simulink model "torqueControlBalancing"  (Simulink 9.1)
settings: Solver=FixedStepDiscrete  StartTime=0.0  StopTime="Config.SIMULATION_TIME "  FixedStep=Config.tStep  RelTol=1e-3  EnableMultiTasking=on
PostLoadFcn:
  | %% Try to open the static GUI and try to adjust it
  | try
  | 
  |     staticGUI = simulinkStaticGUI;
  | 
  | end
InitFcn:
  | %% initialize the simulation
  | cd(fileparts(which(bdroot)));
  | initTorqueControlBalancing;
  | 
  | %% Try to edit the GUI (the user may have already closed it)
  | try
  | 
  |     %% Update Start Button
  |     set(sl_synch_handles.startButton,'Backgroundcolor',[0.0,1.0,0.0]);
  |     set(sl_synch_handles.startButton,'Enable','on');
  | 
  | end
StartFcn:
  | %% Try to edit the GUI (the user may have already closed it)
  | try
  | 
  |     %% Update Start Button
  |     set(sl_synch_handles.startButton,'Backgroundcolor',[0.8,0.8,0.8]);
  |     set(sl_synch_handles.startButton,'Enable','off');
  | 
  |     %% Update Compile Button
  |     set(sl_synch_handles.compileButton,'Backgroundcolor',[0.8,0.8,0.8]);
  |     set(sl_synch_handles.compileButton,'Enable','off');
  | 
  |     %% Update Exit Button
  |     set(sl_synch_handles.exitButton,'Backgroundcolor',[0.8,0.8,0.8]);
  |     set(sl_synch_handles.exitButton,'Enable','off');
  | 
  | end
StopFcn:
  | %% stop the simulation
  | cd(fileparts(which(bdroot)));
  | stopTorqueControlBalancing;
  | 
  | %% Try to edit the GUI (the user may have already closed it)
  | try
  | 
  |     %% Update Compile Button
  |     set(sl_synch_handles.compileButton,'Backgroundcolor',[1.0,0.6,0.0]);
  |     set(sl_synch_handles.compileButton,'Enable','on');
  | 
  |     %% Update Exit Button
  |     set(sl_synch_handles.exitButton,'Backgroundcolor',[0.0,1.0,1.0]);
  |     set(sl_synch_handles.exitButton,'Enable','on');
  | 
  | end
undefined symbols (not defined in the file or in its folder): bVectorConstraints, Config, ConstraintsMatrix, Gain, Reg, ROBOT_DOF, Sat, StateMachine
libraries: WBToolboxLibrary x77
(part 1 of 2)
CloseFcn:
  | %% Try to close the GUI (the user might have already closed it)
  | try
  | 
  |     close(simulinkStaticGUI)
  | 
  | end
settings Model: SuppressorTable=22 serialization::archive 11 0 6 0 0 0 0 0  Creator=daniele  LastModifiedBy=lrapetti
settings DataIOCC: LimitDataPoints=on
settings OptimizationCC: ExpressionDepthLimit=2147483647
settings DebuggingCC: SolverPrmCheckMsg=warning  FcnCallInpInsideContextMsg=warning  AllowSymbolicDim=off  StateNameClashWarn=warning
settings SFSimCC: SimParseCustomCode=off
settings RTWCC: GenCodeOnly=on  TargetLang=C++
settings GRTTargetCC: TargetLangStandard=C++03 (ISO)  GeneratePreprocessorConditionals=Disable all  CombineOutputUpdateFcns=on  MatFileLogging=off  MultiInstanceERTCode=on  CodeInterfacePackaging=C++ class  SupportNonFinite=off  GRTInterface=off
settings CPPComponent: GenerateDestructor=on  GenerateExternalIOAccessMethods=None  ParameterMemberVisibility=private  InternalMemberVisibility=private  GenerateParameterAccessMethods=None  GenerateInternalMemberAccessMethods=None  UseOperatorNewForModelRefRegistration=off

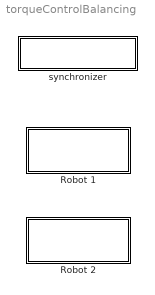
== system torqueControlBalancing ==
  Robot 1 : Subsystem
  Robot 2 : Subsystem
  synchronizer : Subsystem
      mask Display: disp('SYNCHRONIZER')

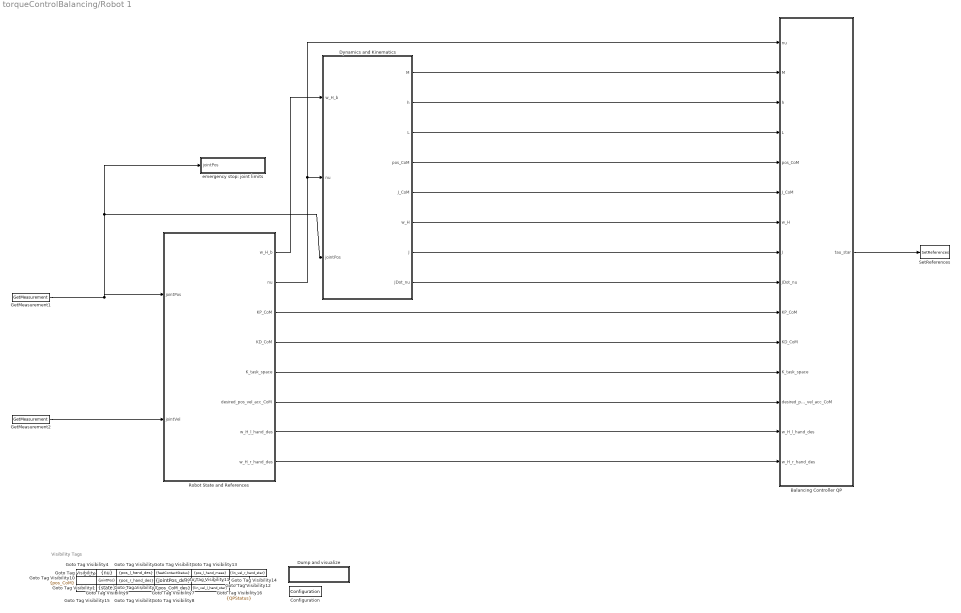
== system torqueControlBalancing/Robot 1 ==
  note: Visibility Tags
  Balancing Controller QP : Subsystem
  Configuration : WBToolboxLibrary/Utilities/Configuration  ConfigSource=Workspace  ConfigObject='WBTConfigRobot_1'
      settings: SourceProductName=WholeBodyToolbox
  Dump and visualize : Subsystem
      mask Display: disp('VISUALIZER')
  Dynamics and Kinematics : Subsystem
  GetMeasurement1 : WBToolboxLibrary/States/GetMeasurement  measuredType=Joints Position
      settings: SourceProductName=WholeBodyToolbox
  GetMeasurement2 : WBToolboxLibrary/States/GetMeasurement  measuredType=Joints Velocity
      settings: SourceProductName=WholeBodyToolbox
  Goto Tag Visibility : GotoTagVisibility  GotoTag=nu
  Goto Tag Visibility1 : GotoTagVisibility  GotoTag=state
  Goto Tag Visibility10 : GotoTagVisibility  GotoTag=pos_CoM
  Goto Tag Visibility11 : GotoTagVisibility  GotoTag=lin_vel_l_hand_star
  Goto Tag Visibility12 : GotoTagVisibility  GotoTag=lin_vel_r_hand_star
  Goto Tag Visibility13 : GotoTagVisibility  GotoTag=pos_l_hand_meas
  Goto Tag Visibility14 : GotoTagVisibility  GotoTag=pos_r_hand_meas
  Goto Tag Visibility15 : GotoTagVisibility  GotoTag=tau_star
  Goto Tag Visibility16 : GotoTagVisibility  GotoTag=QPStatus
  Goto Tag Visibility2 : GotoTagVisibility  GotoTag=pos_l_hand_des
  Goto Tag Visibility3 : GotoTagVisibility  GotoTag=pos_r_hand_des
  Goto Tag Visibility4 : GotoTagVisibility  GotoTag=w_H_b
  Goto Tag Visibility5 : GotoTagVisibility  GotoTag=feetContactStatus
  Goto Tag Visibility6 : GotoTagVisibility  GotoTag=KP_postural_diag
  Goto Tag Visibility7 : GotoTagVisibility  GotoTag=jointPos_des
  Goto Tag Visibility8 : GotoTagVisibility  GotoTag=pos_CoM_des
  Goto Tag Visibility9 : GotoTagVisibility  GotoTag=jointPos
  Robot State and References : Subsystem  Priority=-10
  SetReferences : WBToolboxLibrary/Actuators/SetReferences  controlType=Torque  refSpeed=50  refAcceleration=1000000*(pi/180)
      settings: SourceProductName=WholeBodyToolbox
  emergency stop: joint limits : Subsystem
      mask Display: disp('EMERGENCY STOP')
  wires:
  Robot State and References/3(KP_CoM) -> Balancing Controller QP/10(KP_CoM)
  GetMeasurement2/1 -> Robot State and References/2(jointVel)
  GetMeasurement1/1 -> Dynamics and Kinematics/3(jointPos), emergency stop: joint limits/1(jointPos), Robot State and References/1(jointPos)
  Robot State and References/6(desired_pos_vel_acc_CoM) -> Balancing Controller QP/13(desired_pos_vel_acc_CoM)
  Dynamics and Kinematics/7(J) -> Balancing Controller QP/8(J)
  Dynamics and Kinematics/4(pos_CoM) -> Balancing Controller QP/5(pos_CoM)
  Dynamics and Kinematics/2(h) -> Balancing Controller QP/3(h)
  Robot State and References/1(w_H_b) -> Dynamics and Kinematics/1(w_H_b)
  Dynamics and Kinematics/3(L) -> Balancing Controller QP/4("L ")
  Robot State and References/4(KD_CoM) -> Balancing Controller QP/11(KD_CoM)
  Robot State and References/2(nu) -> Balancing Controller QP/1(nu), Dynamics and Kinematics/2(nu)
  Dynamics and Kinematics/5(J_CoM) -> Balancing Controller QP/6(J_CoM)
  Dynamics and Kinematics/1(M) -> Balancing Controller QP/2(M)
  Dynamics and Kinematics/6(w_H) -> Balancing Controller QP/7(w_H)
  Balancing Controller QP/1("tau_star ") -> SetReferences/1
  Robot State and References/5(K_task_space) -> Balancing Controller QP/12(K_task_space)
  Dynamics and Kinematics/8(JDot_nu) -> Balancing Controller QP/9(JDot_nu)
  Robot State and References/7(w_H_l_hand_des) -> Balancing Controller QP/14(w_H_l_hand_des)
  Robot State and References/8(w_H_r_hand_des) -> Balancing Controller QP/15(w_H_r_hand_des)

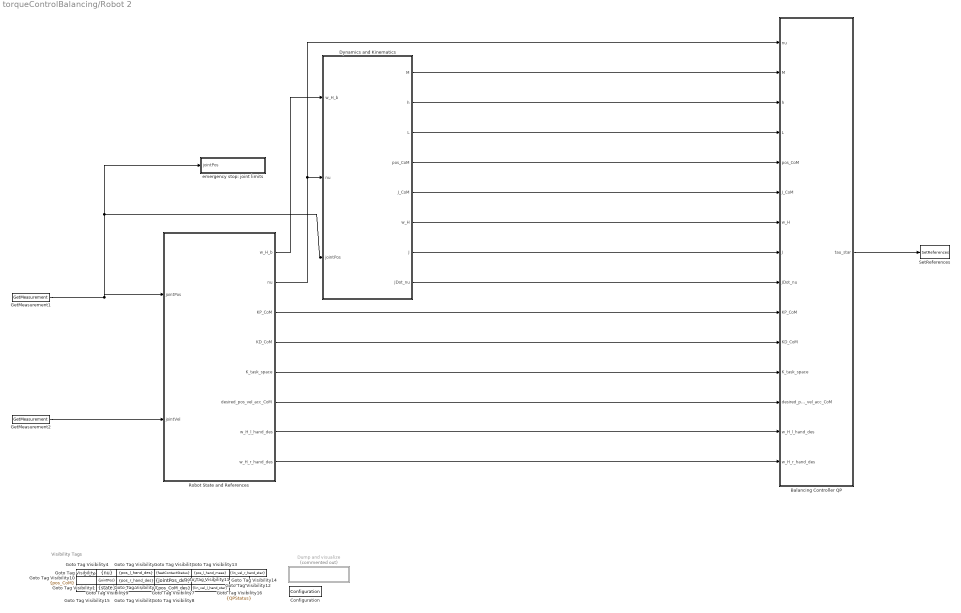
== system torqueControlBalancing/Robot 2 ==
  note: Visibility Tags
  Balancing Controller QP : Subsystem
  Configuration : WBToolboxLibrary/Utilities/Configuration  ConfigSource=Workspace  ConfigObject='WBTConfigRobot_2'
      settings: SourceProductName=WholeBodyToolbox
  Dump and visualize : Subsystem  Commented=on
      mask Display: disp('VISUALIZER')
  Dynamics and Kinematics : Subsystem
  GetMeasurement1 : WBToolboxLibrary/States/GetMeasurement  measuredType=Joints Position
      settings: SourceProductName=WholeBodyToolbox
  GetMeasurement2 : WBToolboxLibrary/States/GetMeasurement  measuredType=Joints Velocity
      settings: SourceProductName=WholeBodyToolbox
  Goto Tag Visibility : GotoTagVisibility  GotoTag=nu
  Goto Tag Visibility1 : GotoTagVisibility  GotoTag=state
  Goto Tag Visibility10 : GotoTagVisibility  GotoTag=pos_CoM
  Goto Tag Visibility11 : GotoTagVisibility  GotoTag=lin_vel_l_hand_star
  Goto Tag Visibility12 : GotoTagVisibility  GotoTag=lin_vel_r_hand_star
  Goto Tag Visibility13 : GotoTagVisibility  GotoTag=pos_l_hand_meas
  Goto Tag Visibility14 : GotoTagVisibility  GotoTag=pos_r_hand_meas
  Goto Tag Visibility15 : GotoTagVisibility  GotoTag=tau_star
  Goto Tag Visibility16 : GotoTagVisibility  GotoTag=QPStatus
  Goto Tag Visibility2 : GotoTagVisibility  GotoTag=pos_l_hand_des
  Goto Tag Visibility3 : GotoTagVisibility  GotoTag=pos_r_hand_des
  Goto Tag Visibility4 : GotoTagVisibility  GotoTag=w_H_b
  Goto Tag Visibility5 : GotoTagVisibility  GotoTag=feetContactStatus
  Goto Tag Visibility6 : GotoTagVisibility  GotoTag=KP_postural_diag
  Goto Tag Visibility7 : GotoTagVisibility  GotoTag=jointPos_des
  Goto Tag Visibility8 : GotoTagVisibility  GotoTag=pos_CoM_des
  Goto Tag Visibility9 : GotoTagVisibility  GotoTag=jointPos
  Robot State and References : Subsystem  Priority=-10
  SetReferences : WBToolboxLibrary/Actuators/SetReferences  controlType=Torque  refSpeed=50  refAcceleration=1000000*(pi/180)
      settings: SourceProductName=WholeBodyToolbox
  emergency stop: joint limits : Subsystem
      mask Display: disp('EMERGENCY STOP')
  wires:
  Robot State and References/3(KP_CoM) -> Balancing Controller QP/10(KP_CoM)
  GetMeasurement2/1 -> Robot State and References/2(jointVel)
  GetMeasurement1/1 -> Dynamics and Kinematics/3(jointPos), emergency stop: joint limits/1(jointPos), Robot State and References/1(jointPos)
  Robot State and References/6(desired_pos_vel_acc_CoM) -> Balancing Controller QP/13(desired_pos_vel_acc_CoM)
  Dynamics and Kinematics/7(J) -> Balancing Controller QP/8(J)
  Dynamics and Kinematics/4(pos_CoM) -> Balancing Controller QP/5(pos_CoM)
  Dynamics and Kinematics/2(h) -> Balancing Controller QP/3(h)
  Robot State and References/1(w_H_b) -> Dynamics and Kinematics/1(w_H_b)
  Dynamics and Kinematics/3(L) -> Balancing Controller QP/4("L ")
  Robot State and References/4(KD_CoM) -> Balancing Controller QP/11(KD_CoM)
  Robot State and References/2(nu) -> Balancing Controller QP/1(nu), Dynamics and Kinematics/2(nu)
  Dynamics and Kinematics/5(J_CoM) -> Balancing Controller QP/6(J_CoM)
  Dynamics and Kinematics/1(M) -> Balancing Controller QP/2(M)
  Dynamics and Kinematics/6(w_H) -> Balancing Controller QP/7(w_H)
  Balancing Controller QP/1("tau_star ") -> SetReferences/1
  Robot State and References/5(K_task_space) -> Balancing Controller QP/12(K_task_space)
  Dynamics and Kinematics/8(JDot_nu) -> Balancing Controller QP/9(JDot_nu)
  Robot State and References/7(w_H_l_hand_des) -> Balancing Controller QP/14(w_H_l_hand_des)
  Robot State and References/8(w_H_r_hand_des) -> Balancing Controller QP/15(w_H_r_hand_des)

== system torqueControlBalancing/synchronizer ==
  GAZEBO_SYNCHRONIZER : Subsystem
  Logical Operator : Logic  Operator=NOT  AllPortsSameDT=off  OutDataTypeStr=boolean
  "ON_GAZEBO " : Constant  Value=Config.ON_GAZEBO
  REAL_TIME_SYNC : Subsystem
  To Workspace : ToWorkspace  VariableName=yarp_time  SaveFormat=Structure With Time  SampleTime=-1
  Yarp Clock : WBToolboxLibrary/Utilities/Yarp Clock
      settings: SourceProductName=WholeBodyToolbox
  wires:
  Logical Operator/1 -> REAL_TIME_SYNC/Enable
  "ON_GAZEBO "/1 -> GAZEBO_SYNCHRONIZER/Enable, Logical Operator/1
  Yarp Clock/1 -> To Workspace/1

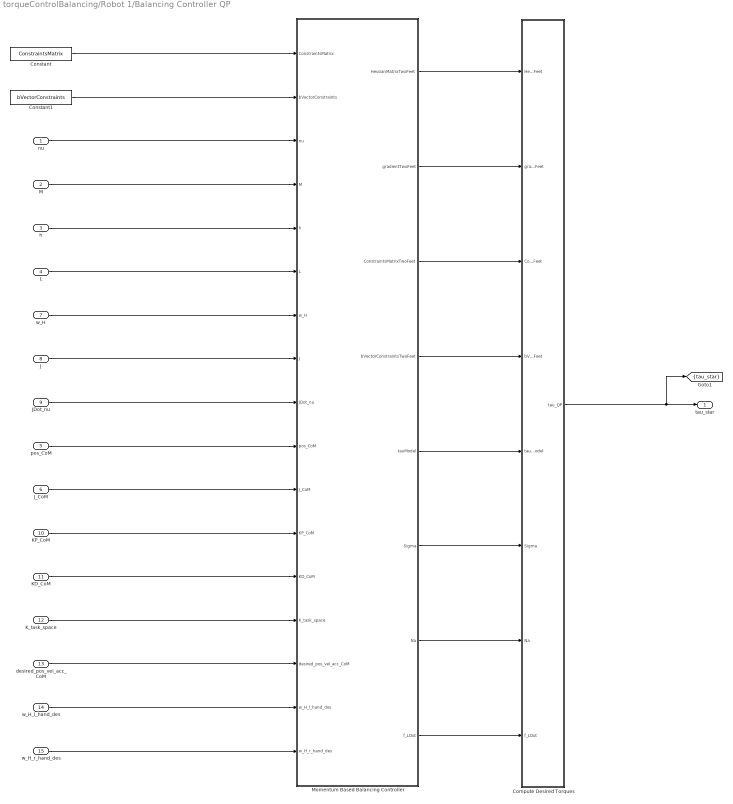
== system torqueControlBalancing/Robot 1/Balancing Controller QP ==
  nu : Inport
  M : Inport  Port=2
  h : Inport  Port=3
  "L " : Inport  Port=4
  pos_CoM : Inport  Port=5
  J_CoM : Inport  Port=6
  w_H : Inport  Port=7
  J : Inport  Port=8
  JDot_nu : Inport  Port=9
  KP_CoM : Inport  Port=10
  KD_CoM : Inport  Port=11
  K_task_space : Inport  Port=12
  desired_pos_vel_acc_CoM : Inport  Port=13
  w_H_l_hand_des : Inport  Port=14
  w_H_r_hand_des : Inport  Port=15
  Compute Desired Torques : Subsystem
  Constant : Constant  Value=ConstraintsMatrix
  Constant1 : Constant  Value=bVectorConstraints
  "Momentum Based Balancing Controller " : MATLAB Function  TreatAsAtomicUnit=on
  "tau_star " : Outport
  tag scope: tau_star=scoped
  wires:
  Compute Desired Torques/1(tau_QP) -> [tau_star], "tau_star "/1
  Constant1/1 -> "Momentum Based Balancing Controller "/2(bVectorConstraints)
  Constant/1 -> "Momentum Based Balancing Controller "/1(ConstraintsMatrix)
  nu/1 -> "Momentum Based Balancing Controller "/3(nu)
  M/1 -> "Momentum Based Balancing Controller "/4(M)
  h/1 -> "Momentum Based Balancing Controller "/5(h)
  "L "/1 -> "Momentum Based Balancing Controller "/6(L)
  pos_CoM/1 -> "Momentum Based Balancing Controller "/10(pos_CoM)
  J_CoM/1 -> "Momentum Based Balancing Controller "/11(J_CoM)
  desired_pos_vel_acc_CoM/1 -> "Momentum Based Balancing Controller "/15(desired_pos_vel_acc_CoM)
  KP_CoM/1 -> "Momentum Based Balancing Controller "/12(KP_CoM)
  KD_CoM/1 -> "Momentum Based Balancing Controller "/13(KD_CoM)
  "Momentum Based Balancing Controller "/1(HessianMatrixTwoFeet) -> Compute Desired Torques/1(HessianMatrixTwoFeet)
  "Momentum Based Balancing Controller "/2(gradientTwoFeet) -> Compute Desired Torques/2(gradientTwoFeet)
  "Momentum Based Balancing Controller "/3(ConstraintsMatrixTwoFeet) -> Compute Desired Torques/3(ConstraintsMatrixTwoFeet)
  "Momentum Based Balancing Controller "/4(bVectorConstraintsTwoFeet) -> Compute Desired Torques/4(bVectorConstraintsTwoFeet)
  "Momentum Based Balancing Controller "/5(tauModel) -> Compute Desired Torques/5(tauModel)
  "Momentum Based Balancing Controller "/6(Sigma) -> Compute Desired Torques/6(Sigma)
  "Momentum Based Balancing Controller "/7(Na) -> Compute Desired Torques/7(Na)
  "Momentum Based Balancing Controller "/8(f_LDot) -> Compute Desired Torques/8(f_LDot)
  w_H/1 -> "Momentum Based Balancing Controller "/7(w_H)
  J/1 -> "Momentum Based Balancing Controller "/8(J)
  K_task_space/1 -> "Momentum Based Balancing Controller "/14(K_task_space)
  JDot_nu/1 -> "Momentum Based Balancing Controller "/9(JDot_nu)
  w_H_l_hand_des/1 -> "Momentum Based Balancing Controller "/16(w_H_l_hand_des)
  w_H_r_hand_des/1 -> "Momentum Based Balancing Controller "/17(w_H_r_hand_des)

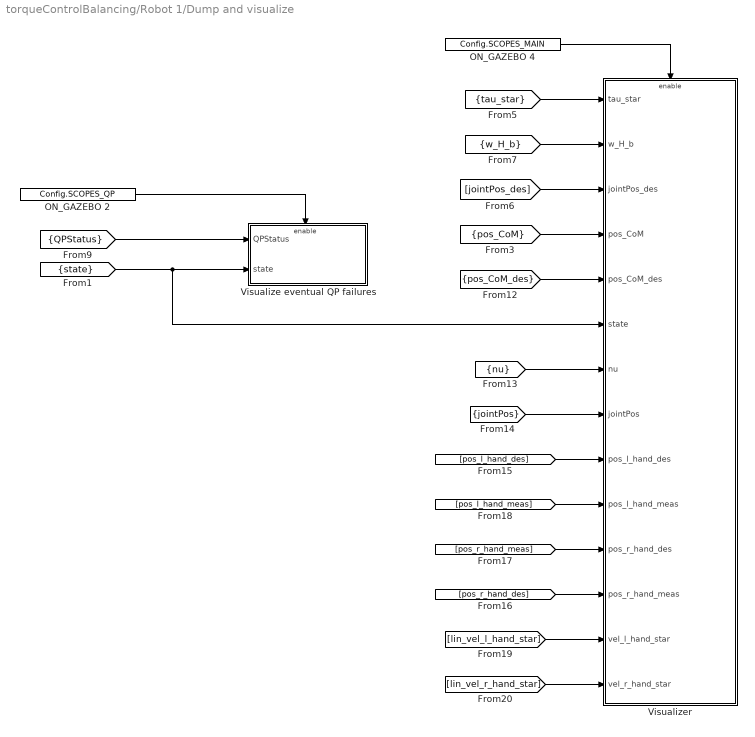
== system torqueControlBalancing/Robot 1/Dump and visualize ==
  ON_GAZEBO 2 : Constant  Value=Config.SCOPES_QP
  ON_GAZEBO 4 : Constant  Value=Config.SCOPES_MAIN
  Visualize eventual QP failures : Subsystem
  Visualizer : Subsystem
  wires:
  ON_GAZEBO 4/1 -> Visualizer/Enable
  [state] -> Visualize eventual QP failures/2(state), Visualizer/6(state)
  [w_H_b] -> Visualizer/2(w_H_b)
  [tau_star] -> Visualizer/1(tau_star)
  [pos_CoM_des] -> Visualizer/5(pos_CoM_des)
  ON_GAZEBO 2/1 -> Visualize eventual QP failures/Enable
  [QPStatus] -> Visualize eventual QP failures/1(QPStatus)
  [jointPos_des] -> Visualizer/3(jointPos_des)
  [pos_CoM] -> Visualizer/4(pos_CoM)
  [nu] -> Visualizer/7(nu)
  [jointPos] -> Visualizer/8(jointPos)
  [pos_l_hand_des] -> Visualizer/9(pos_l_hand_des)
  [pos_l_hand_meas] -> Visualizer/10(pos_l_hand_meas)
  [pos_r_hand_meas] -> Visualizer/11(pos_r_hand_des)
  [pos_r_hand_des] -> Visualizer/12(pos_r_hand_meas)
  [lin_vel_l_hand_star] -> Visualizer/13(vel_l_hand_star)
  [lin_vel_r_hand_star] -> Visualizer/14(vel_r_hand_star)

== system torqueControlBalancing/Robot 1/Dynamics and Kinematics ==
  w_H_b : Inport
  nu : Inport  Port=2
  jointPos : Inport  Port=3
  Concatenate J : Concatenate  NumInputs=4  Mode=Multidimensional array
  Concatenate JDot_nu : Concatenate  NumInputs=4  Mode=Multidimensional array
  Concatenate w_H : Concatenate  NumInputs=4  Mode=Multidimensional array
  Dynamics : Subsystem
  Kinematics : Subsystem
  M : Outport
  h : Outport  Port=2
  L : Outport  Port=3
  pos_CoM : Outport  Port=4
  J_CoM : Outport  Port=5
  w_H : Outport  Port=6
  J : Outport  Port=7
  JDot_nu : Outport  Port=8
  wires:
  w_H_b/1 -> Kinematics/3(w_H_b), Dynamics/1(w_H_b)
  jointPos/1 -> Dynamics/2(jointPos), Kinematics/2(jointPos)
  nu/1 -> Dynamics/3(nu), Kinematics/1(nu)
  Dynamics/1(M) -> M/1
  Dynamics/2(h) -> h/1
  Dynamics/3(L) -> L/1
  Kinematics/11(JDot_l_sole_nu) -> Concatenate JDot_nu/1
  Kinematics/12(JDot_r_sole_nu) -> Concatenate JDot_nu/2
  Kinematics/8(J_r_sole) -> Concatenate J/2
  Kinematics/7(J_l_sole) -> Concatenate J/1
  Kinematics/2(J_CoM) -> J_CoM/1
  Kinematics/1(pos_CoM) -> pos_CoM/1
  Kinematics/9(J_l_hand) -> Concatenate J/3
  Kinematics/10(J_r_hand) -> Concatenate J/4
  Kinematics/6(w_H_r_hand) -> Concatenate w_H/4
  Kinematics/5(w_H_l_hand) -> Concatenate w_H/3
  Kinematics/4(w_H_r_sole) -> Concatenate w_H/2
  Kinematics/3(w_H_l_sole) -> Concatenate w_H/1
  Concatenate w_H/1 -> w_H/1
  Concatenate J/1 -> J/1
  Kinematics/13(JDot_l_hand_nu) -> Concatenate JDot_nu/3
  Kinematics/14(JDot_r_hand_nu) -> Concatenate JDot_nu/4
  Concatenate JDot_nu/1 -> JDot_nu/1

== system torqueControlBalancing/Robot 1/Robot State and References ==
  jointPos : Inport
  jointVel : Inport  Port=2
  Compute State Velocity : Subsystem
  Compute base to fixed link transform : Subsystem
  State Machine : Subsystem  Priority=-100
  Update Gains and References : Subsystem
  w_H_b : Outport
  nu : Outport  Port=2
  KP_CoM : Outport  Port=3
  KD_CoM : Outport  Port=4
  K_task_space : Outport  Port=5
  desired_pos_vel_acc_CoM : Outport  Port=6
  w_H_l_hand_des : Outport  Port=7
  w_H_r_hand_des : Outport  Port=8
  tag scope: nu=scoped, state=scoped
  wires:
  Compute base to fixed link transform/1(fixed_l_sole_H_b) -> State Machine/2(fixed_l_sole_H_b)
  State Machine/1(w_H_b) -> w_H_b/1, Compute State Velocity/3(w_H_b)
  State Machine/2(pos_CoM_des) -> Update Gains and References/1(pos_CoM_des)
  State Machine/3(KP_CoM_diag) -> Update Gains and References/2(KP_CoM_diag)
  State Machine/4(KD_CoM_diag) -> Update Gains and References/3(KD_CoM_diag)
  State Machine/5(smoothingTime_CoM) -> Update Gains and References/4(smoothingTime_CoM)
  Compute State Velocity/1(nu) -> [nu], nu/1
  Update Gains and References/1(KP_CoM) -> KP_CoM/1
  Update Gains and References/2(KD_CoM) -> KD_CoM/1
  Update Gains and References/3(desired_pos_vel_acc_CoM) -> desired_pos_vel_acc_CoM/1
  jointPos/1 -> Compute base to fixed link transform/1(jointPos), Compute State Velocity/1(jointPos), State Machine/1(jointPos)
  jointVel/1 -> Compute State Velocity/2(jointVel)
  State Machine/9(K_task_space) -> K_task_space/1
  State Machine/6(state) -> [state]
  State Machine/7(w_H_l_hand_des) -> w_H_l_hand_des/1
  State Machine/8(w_H_r_hand_des) -> w_H_r_hand_des/1

== system torqueControlBalancing/Robot 1/emergency stop: joint limits ==
  jointPos : Inport
  ON_GAZEBO 1 : Constant  Value=Config.EMERGENCY_STOP_WITH_JOINTS_LIMITS
  ON_GAZEBO 2 : Constant  Value=Config.EMERGENCY_STOP_WITH_ENCODER_SPIKES
  STOP IF JOINTS HIT THE LIMITS : Subsystem
  STOP IF THERE ARE SPIKES IN THE ENCODERS : Subsystem
  wires:
  ON_GAZEBO 1/1 -> STOP IF JOINTS HIT THE LIMITS/Enable
  jointPos/1 -> STOP IF THERE ARE SPIKES IN THE ENCODERS/1(jointPos), STOP IF JOINTS HIT THE LIMITS/1(jointPos)
  ON_GAZEBO 2/1 -> STOP IF THERE ARE SPIKES IN THE ENCODERS/Enable

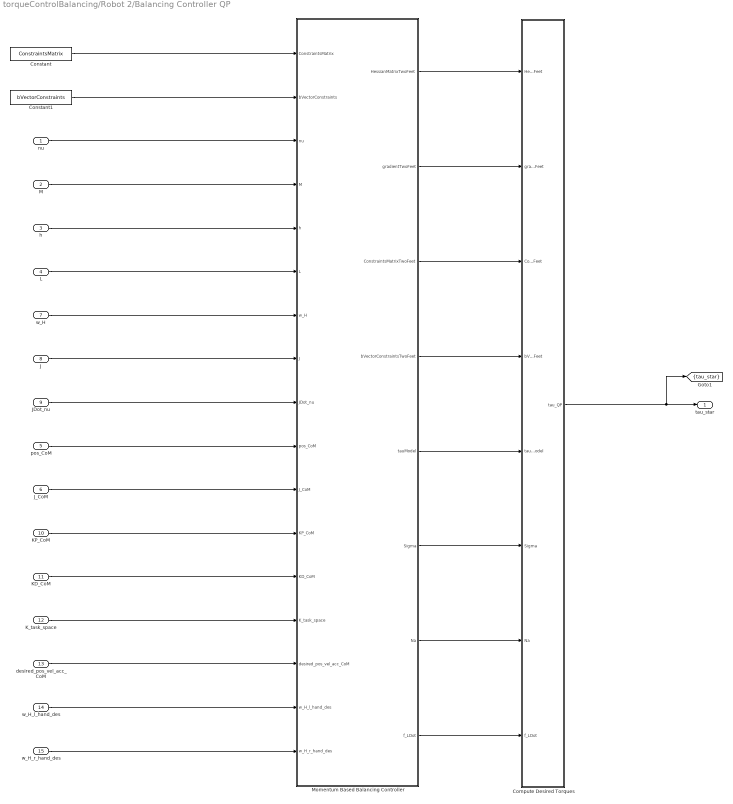
== system torqueControlBalancing/Robot 2/Balancing Controller QP ==
  nu : Inport
  M : Inport  Port=2
  h : Inport  Port=3
  "L " : Inport  Port=4
  pos_CoM : Inport  Port=5
  J_CoM : Inport  Port=6
  w_H : Inport  Port=7
  J : Inport  Port=8
  JDot_nu : Inport  Port=9
  KP_CoM : Inport  Port=10
  KD_CoM : Inport  Port=11
  K_task_space : Inport  Port=12
  desired_pos_vel_acc_CoM : Inport  Port=13
  w_H_l_hand_des : Inport  Port=14
  w_H_r_hand_des : Inport  Port=15
  Compute Desired Torques : Subsystem
  Constant : Constant  Value=ConstraintsMatrix
  Constant1 : Constant  Value=bVectorConstraints
  "Momentum Based Balancing Controller " : MATLAB Function  TreatAsAtomicUnit=on
  "tau_star " : Outport
  tag scope: tau_star=scoped
  wires:
  Compute Desired Torques/1(tau_QP) -> [tau_star], "tau_star "/1
  Constant1/1 -> "Momentum Based Balancing Controller "/2(bVectorConstraints)
  Constant/1 -> "Momentum Based Balancing Controller "/1(ConstraintsMatrix)
  nu/1 -> "Momentum Based Balancing Controller "/3(nu)
  M/1 -> "Momentum Based Balancing Controller "/4(M)
  h/1 -> "Momentum Based Balancing Controller "/5(h)
  "L "/1 -> "Momentum Based Balancing Controller "/6(L)
  pos_CoM/1 -> "Momentum Based Balancing Controller "/10(pos_CoM)
  J_CoM/1 -> "Momentum Based Balancing Controller "/11(J_CoM)
  desired_pos_vel_acc_CoM/1 -> "Momentum Based Balancing Controller "/15(desired_pos_vel_acc_CoM)
  KP_CoM/1 -> "Momentum Based Balancing Controller "/12(KP_CoM)
  KD_CoM/1 -> "Momentum Based Balancing Controller "/13(KD_CoM)
  "Momentum Based Balancing Controller "/1(HessianMatrixTwoFeet) -> Compute Desired Torques/1(HessianMatrixTwoFeet)
  "Momentum Based Balancing Controller "/2(gradientTwoFeet) -> Compute Desired Torques/2(gradientTwoFeet)
  "Momentum Based Balancing Controller "/3(ConstraintsMatrixTwoFeet) -> Compute Desired Torques/3(ConstraintsMatrixTwoFeet)
  "Momentum Based Balancing Controller "/4(bVectorConstraintsTwoFeet) -> Compute Desired Torques/4(bVectorConstraintsTwoFeet)
  "Momentum Based Balancing Controller "/5(tauModel) -> Compute Desired Torques/5(tauModel)
  "Momentum Based Balancing Controller "/6(Sigma) -> Compute Desired Torques/6(Sigma)
  "Momentum Based Balancing Controller "/7(Na) -> Compute Desired Torques/7(Na)
  "Momentum Based Balancing Controller "/8(f_LDot) -> Compute Desired Torques/8(f_LDot)
  w_H/1 -> "Momentum Based Balancing Controller "/7(w_H)
  J/1 -> "Momentum Based Balancing Controller "/8(J)
  K_task_space/1 -> "Momentum Based Balancing Controller "/14(K_task_space)
  JDot_nu/1 -> "Momentum Based Balancing Controller "/9(JDot_nu)
  w_H_l_hand_des/1 -> "Momentum Based Balancing Controller "/16(w_H_l_hand_des)
  w_H_r_hand_des/1 -> "Momentum Based Balancing Controller "/17(w_H_r_hand_des)

== system torqueControlBalancing/Robot 2/Dump and visualize ==
  ON_GAZEBO 2 : Constant  Value=Config.SCOPES_QP
  ON_GAZEBO 4 : Constant  Value=Config.SCOPES_MAIN
  Visualize eventual QP failures : Subsystem
  Visualizer : Subsystem
  wires:
  ON_GAZEBO 4/1 -> Visualizer/Enable
  [state] -> Visualize eventual QP failures/2(state), Visualizer/6(state)
  [w_H_b] -> Visualizer/2(w_H_b)
  [tau_star] -> Visualizer/1(tau_star)
  [pos_CoM_des] -> Visualizer/5(pos_CoM_des)
  ON_GAZEBO 2/1 -> Visualize eventual QP failures/Enable
  [QPStatus] -> Visualize eventual QP failures/1(QPStatus)
  [jointPos_des] -> Visualizer/3(jointPos_des)
  [pos_CoM] -> Visualizer/4(pos_CoM)
  [nu] -> Visualizer/7(nu)
  [jointPos] -> Visualizer/8(jointPos)
  [pos_l_hand_des] -> Visualizer/9(pos_l_hand_des)
  [pos_l_hand_meas] -> Visualizer/10(pos_l_hand_meas)
  [pos_r_hand_meas] -> Visualizer/11(pos_r_hand_des)
  [pos_r_hand_des] -> Visualizer/12(pos_r_hand_meas)
  [lin_vel_l_hand_star] -> Visualizer/13(vel_l_hand_star)
  [lin_vel_r_hand_star] -> Visualizer/14(vel_r_hand_star)

== system torqueControlBalancing/Robot 2/Dynamics and Kinematics ==
  w_H_b : Inport
  nu : Inport  Port=2
  jointPos : Inport  Port=3
  Concatenate J : Concatenate  NumInputs=4  Mode=Multidimensional array
  Concatenate JDot_nu : Concatenate  NumInputs=4  Mode=Multidimensional array
  Concatenate w_H : Concatenate  NumInputs=4  Mode=Multidimensional array
  Dynamics : Subsystem
  Kinematics : Subsystem
  M : Outport
  h : Outport  Port=2
  L : Outport  Port=3
  pos_CoM : Outport  Port=4
  J_CoM : Outport  Port=5
  w_H : Outport  Port=6
  J : Outport  Port=7
  JDot_nu : Outport  Port=8
  wires:
  w_H_b/1 -> Kinematics/3(w_H_b), Dynamics/1(w_H_b)
  jointPos/1 -> Dynamics/2(jointPos), Kinematics/2(jointPos)
  nu/1 -> Dynamics/3(nu), Kinematics/1(nu)
  Dynamics/1(M) -> M/1
  Dynamics/2(h) -> h/1
  Dynamics/3(L) -> L/1
  Kinematics/11(JDot_l_sole_nu) -> Concatenate JDot_nu/1
  Kinematics/12(JDot_r_sole_nu) -> Concatenate JDot_nu/2
  Kinematics/8(J_r_sole) -> Concatenate J/2
  Kinematics/7(J_l_sole) -> Concatenate J/1
  Kinematics/2(J_CoM) -> J_CoM/1
  Kinematics/1(pos_CoM) -> pos_CoM/1
  Kinematics/9(J_l_hand) -> Concatenate J/3
  Kinematics/10(J_r_hand) -> Concatenate J/4
  Kinematics/6(w_H_r_hand) -> Concatenate w_H/4
  Kinematics/5(w_H_l_hand) -> Concatenate w_H/3
  Kinematics/4(w_H_r_sole) -> Concatenate w_H/2
  Kinematics/3(w_H_l_sole) -> Concatenate w_H/1
  Concatenate w_H/1 -> w_H/1
  Concatenate J/1 -> J/1
  Kinematics/13(JDot_l_hand_nu) -> Concatenate JDot_nu/3
  Kinematics/14(JDot_r_hand_nu) -> Concatenate JDot_nu/4
  Concatenate JDot_nu/1 -> JDot_nu/1

== system torqueControlBalancing/Robot 2/Robot State and References ==
  jointPos : Inport
  jointVel : Inport  Port=2
  Compute State Velocity : Subsystem
  Compute base to fixed link transform : Subsystem
  State Machine : Subsystem  Priority=-100
  Update Gains and References : Subsystem
  w_H_b : Outport
  nu : Outport  Port=2
  KP_CoM : Outport  Port=3
  KD_CoM : Outport  Port=4
  K_task_space : Outport  Port=5
  desired_pos_vel_acc_CoM : Outport  Port=6
  w_H_l_hand_des : Outport  Port=7
  w_H_r_hand_des : Outport  Port=8
  tag scope: nu=scoped, state=scoped
  wires:
  Compute base to fixed link transform/1(fixed_l_sole_H_b) -> State Machine/2(fixed_l_sole_H_b)
  State Machine/1(w_H_b) -> w_H_b/1, Compute State Velocity/3(w_H_b)
  State Machine/2(pos_CoM_des) -> Update Gains and References/1(pos_CoM_des)
  State Machine/3(KP_CoM_diag) -> Update Gains and References/2(KP_CoM_diag)
  State Machine/4(KD_CoM_diag) -> Update Gains and References/3(KD_CoM_diag)
  State Machine/5(smoothingTime_CoM) -> Update Gains and References/4(smoothingTime_CoM)
  Compute State Velocity/1(nu) -> [nu], nu/1
  Update Gains and References/1(KP_CoM) -> KP_CoM/1
  Update Gains and References/2(KD_CoM) -> KD_CoM/1
  Update Gains and References/3(desired_pos_vel_acc_CoM) -> desired_pos_vel_acc_CoM/1
  jointPos/1 -> Compute base to fixed link transform/1(jointPos), Compute State Velocity/1(jointPos), State Machine/1(jointPos)
  jointVel/1 -> Compute State Velocity/2(jointVel)
  State Machine/9(K_task_space) -> K_task_space/1
  State Machine/6(state) -> [state]
  State Machine/7(w_H_l_hand_des) -> w_H_l_hand_des/1
  State Machine/8(w_H_r_hand_des) -> w_H_r_hand_des/1

== system torqueControlBalancing/Robot 2/emergency stop: joint limits ==
  jointPos : Inport
  ON_GAZEBO 1 : Constant  Value=Config.EMERGENCY_STOP_WITH_JOINTS_LIMITS
  ON_GAZEBO 2 : Constant  Value=Config.EMERGENCY_STOP_WITH_ENCODER_SPIKES
  STOP IF JOINTS HIT THE LIMITS : Subsystem
  STOP IF THERE ARE SPIKES IN THE ENCODERS : Subsystem
  wires:
  ON_GAZEBO 1/1 -> STOP IF JOINTS HIT THE LIMITS/Enable
  jointPos/1 -> STOP IF THERE ARE SPIKES IN THE ENCODERS/1(jointPos), STOP IF JOINTS HIT THE LIMITS/1(jointPos)
  ON_GAZEBO 2/1 -> STOP IF THERE ARE SPIKES IN THE ENCODERS/Enable

== system torqueControlBalancing/synchronizer/GAZEBO_SYNCHRONIZER ==
  Enable : EnablePort
  Simulator Synchronizer : WBToolboxLibrary/Utilities/Simulator Synchronizer  period=Config.tStep  serverPortName='/clock/rpc'  clientPortName='/WBT_synchronizer/rpc:o'
      settings: SourceProductName=WholeBodyToolbox

== system torqueControlBalancing/synchronizer/REAL_TIME_SYNC ==
  Enable : EnablePort
  Real Time Synchronizer : WBToolboxLibrary/Utilities/Real Time Synchronizer  period=Config.tStep
      settings: SourceProductName=WholeBodyToolbox

== system torqueControlBalancing/Robot 1/Balancing Controller QP/Compute Desired Torques ==
  HessianMatrixTwoFeet : Inport
  gradientTwoFeet : Inport  Port=2
  ConstraintsMatrixTwoFeet : Inport  Port=3
  bVectorConstraintsTwoFeet : Inport  Port=4
  tauModel : Inport  Port=5
  Sigma : Inport  Port=6
  Na : Inport  Port=7
  f_LDot : Inport  Port=8
  Add : Sum
  Add1 : Sum
  Product1 : Product  Multiplication=Matrix(*)
  Product2 : Product  Multiplication=Matrix(*)
  QPSolver : Subsystem
  tau_QP : Outport
  wires:
  Na/1 -> Product2/1
  Product1/1 -> Add/2
  tauModel/1 -> Add/1
  Add/1 -> tau_QP/1
  Add1/1 -> Product1/2
  f_LDot/1 -> Add1/1
  Product2/1 -> Add1/2
  Sigma/1 -> Product1/1
  QPSolver/1(f_0_twoFeet) -> Product2/2
  ConstraintsMatrixTwoFeet/1 -> QPSolver/3(ConstraintsMatrixTwoFeet)
  gradientTwoFeet/1 -> QPSolver/2(gradientTwoFeet)
  HessianMatrixTwoFeet/1 -> QPSolver/1(HessianMatrixTwoFeet)
  bVectorConstraintsTwoFeet/1 -> QPSolver/4(bVectorConstraintsTwoFeet)

== system torqueControlBalancing/Robot 1/Dump and visualize/Visualize eventual QP failures ==
  QPStatus : Inport
  state : Inport  Port=2
  Enable : EnablePort
  QP status (0: no failure) : Scope  NumInputPorts=2
  wires:
  QPStatus/1 -> QP status (0: no failure)/1
  state/1 -> QP status (0: no failure)/2

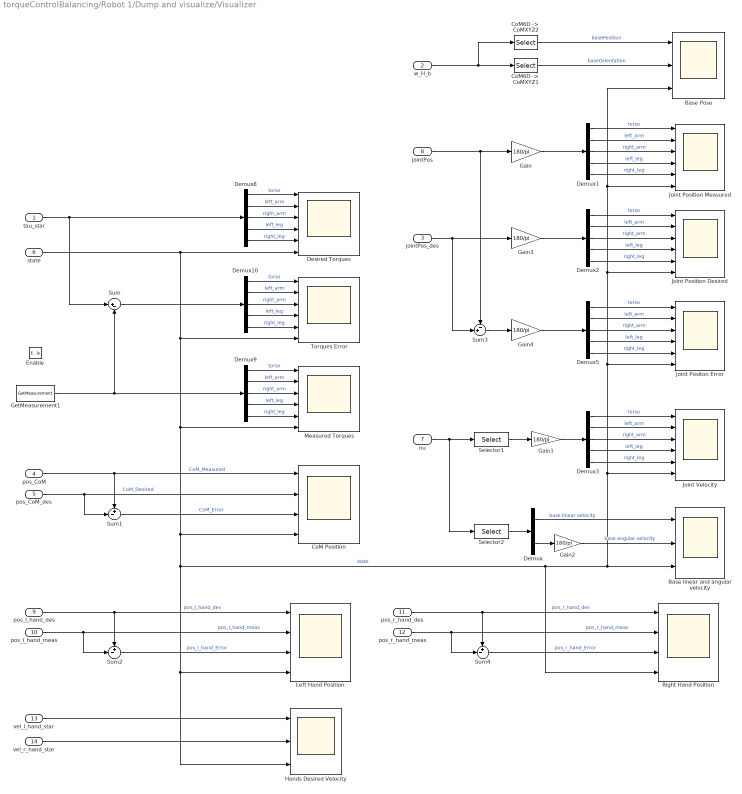
== system torqueControlBalancing/Robot 1/Dump and visualize/Visualizer ==
  tau_star : Inport
  w_H_b : Inport  Port=2
  jointPos_des : Inport  Port=3
  pos_CoM : Inport  Port=4
  pos_CoM_des : Inport  Port=5
  state : Inport  Port=6
  nu : Inport  Port=7
  jointPos : Inport  Port=8
  pos_l_hand_des : Inport  Port=9
  pos_l_hand_meas : Inport  Port=10
  pos_r_hand_des : Inport  Port=11
  pos_r_hand_meas : Inport  Port=12
  vel_l_hand_star : Inport  Port=13
  vel_r_hand_star : Inport  Port=14
  Enable : EnablePort
  Base Pose : Scope  NumInputPorts=3
  Base linear and angular velocity : Scope  NumInputPorts=3
  CoM Position : Scope  NumInputPorts=4
  "CoM6D ->  CoMXYZ1" : Selector  NumberOfDimensions=2  InputPortWidth=7  IndexOptions=Index vector (dialog),Index vector (dialog)  Indices=[1 2 3],[1 2 3]  OutputSizes=1,1
  "CoM6D ->  CoMXYZ2" : Selector  NumberOfDimensions=2  InputPortWidth=7  IndexOptions=Index vector (dialog),Index vector (dialog)  Indices=[1 2 3],[4]  OutputSizes=1,1
  Demux : Demux  Outputs=2
  Demux{1..3,5,8..10} (7 alike) : Demux  Outputs=Config.numOfJointsForEachControlboard
  Desired Torques : Scope  NumInputPorts=6
  Gain{,1..4} (5 alike) : Gain  Gain=180/pi
  GetMeasurement1 : WBToolboxLibrary/States/GetMeasurement  measuredType=Joints Torque
      settings: SourceProductName=WholeBodyToolbox
  Hands Desired Velocity : Scope  NumInputPorts=3
  Joint Position Desired : Scope  NumInputPorts=6
  Joint Position Measured : Scope  NumInputPorts=6
  Joint Positon Error : Scope  NumInputPorts=6
  Joint Velocity : Scope  NumInputPorts=6
  Left Hand Position : Scope  NumInputPorts=4
  Measured Torques : Scope  NumInputPorts=6
  Right Hand Position : Scope  NumInputPorts=4
  Selector1 : Selector  InputPortWidth=6+ROBOT_DOF  IndexOptions=Index vector (dialog)  Indices=[7:6+ROBOT_DOF]  OutputSizes=1
  Selector2 : Selector  InputPortWidth=6+ROBOT_DOF  IndexOptions=Index vector (dialog)  Indices=[1:6]  OutputSizes=1
  Sum : Sum  Inputs=|+-
  Sum1 : Sum  Inputs=+-|
  Sum2 : Sum  Inputs=+-|
  Sum3 : Sum  Inputs=-+|
  Sum4 : Sum  Inputs=+-|
  Torques Error : Scope  NumInputPorts=6
  wires:
  pos_CoM/1 -> Sum1/1, CoM Position/1  "CoM_Measured"
  Gain/1 -> Demux1/1
  jointPos/1 -> Gain/1, Sum3/1
  Demux1/5 -> Joint Position Measured/5  "right_leg"
  Demux1/1 -> Joint Position Measured/1  "torso"
  Demux1/2 -> Joint Position Measured/2  "left_arm"
  Demux1/4 -> Joint Position Measured/4  "left_leg"
  Demux1/3 -> Joint Position Measured/3  "right_arm"
  GetMeasurement1/1 -> Sum/2, Demux9/1
  Demux8/5 -> Desired Torques/5  "right_leg"
  Demux8/1 -> Desired Torques/1  "torso"
  Demux8/2 -> Desired Torques/2  "left_arm"
  Demux8/4 -> Desired Torques/4  "left_leg"
  Demux8/3 -> Desired Torques/3  "right_arm"
  Demux10/5 -> Torques Error/5  "right_leg"
  Demux10/1 -> Torques Error/1  "torso"
  Demux10/2 -> Torques Error/2  "left_arm"
  Demux10/4 -> Torques Error/4  "left_leg"
  Demux10/3 -> Torques Error/3  "right_arm"
  Sum/1 -> Demux10/1
  Demux9/5 -> Measured Torques/5  "right_leg"
  Demux9/1 -> Measured Torques/1  "torso"
  Demux9/2 -> Measured Torques/2  "left_arm"
  Demux9/4 -> Measured Torques/4  "left_leg"
  Demux9/3 -> Measured Torques/3  "right_arm"
  jointPos_des/1 -> Sum3/2, Gain3/1
  Gain3/1 -> Demux2/1
  Demux2/5 -> Joint Position Desired/5  "right_leg"
  Demux2/1 -> Joint Position Desired/1  "torso"
  Demux2/2 -> Joint Position Desired/2  "left_arm"
  Demux2/4 -> Joint Position Desired/4  "left_leg"
  Demux2/3 -> Joint Position Desired/3  "right_arm"
  Gain4/1 -> Demux5/1
  Demux5/5 -> Joint Positon Error/5  "right_leg"
  Demux5/1 -> Joint Positon Error/1  "torso"
  Demux5/2 -> Joint Positon Error/2  "left_arm"
  Demux5/4 -> Joint Positon Error/4  "left_leg"
  Demux5/3 -> Joint Positon Error/3  "right_arm"
  Sum3/1 -> Gain4/1
  pos_CoM_des/1 -> Sum1/2, CoM Position/2  "CoM_Desired"
  w_H_b/1 -> "CoM6D ->  CoMXYZ2"/1, "CoM6D ->  CoMXYZ1"/1
  "CoM6D ->  CoMXYZ2"/1 -> Base Pose/1  "basePosition"
  "CoM6D ->  CoMXYZ1"/1 -> Base Pose/2  "baseOrientation"
  tau_star/1 -> Sum/1, Demux8/1
  nu/1 -> Selector1/1, Selector2/1
  Selector2/1 -> Demux/1
  Gain1/1 -> Demux3/1
  Demux/1 -> Base linear and angular velocity/1  "base linear velocity"
  Gain2/1 -> Base linear and angular velocity/2  "base angular velocity"
  Demux3/3 -> Joint Velocity/3  "right_arm"
  Demux3/5 -> Joint Velocity/5  "right_leg"
  Selector1/1 -> Gain1/1
  Demux3/1 -> Joint Velocity/1  "torso"
  Demux3/2 -> Joint Velocity/2  "left_arm"
  Demux3/4 -> Joint Velocity/4  "left_leg"
  Demux/2 -> Gain2/1
  Sum1/1 -> CoM Position/3  "CoM_Error"
  pos_l_hand_des/1 -> Left Hand Position/1, Sum2/1  "pos_l_hand_des"
  pos_l_hand_meas/1 -> Sum2/2, Left Hand Position/2  "pos_l_hand_meas"
  Sum2/1 -> Left Hand Position/3  "pos_l_hand_Error"
  pos_r_hand_meas/1 -> Sum4/2, Right Hand Position/2  "pos_r_hand_meas"
  pos_r_hand_des/1 -> Right Hand Position/1, Sum4/1  "pos_r_hand_des"
  state/1 -> Left Hand Position/4, Hands Desired Velocity/3, Right Hand Position/4, Base linear and angular velocity/3, Joint Velocity/6, Joint Positon Error/6, Joint Position Desired/6, Base Pose/3, Joint Position Measured/6, CoM Position/4, Measured Torques/6, Torques Error/6, Desired Torques/6  "state"
  Sum4/1 -> Right Hand Position/3  "pos_r_hand_Error"
  vel_l_hand_star/1 -> Hands Desired Velocity/1
  vel_r_hand_star/1 -> Hands Desired Velocity/2

== system torqueControlBalancing/Robot 1/Dynamics and Kinematics/Dynamics ==
  w_H_b : Inport
  jointPos : Inport  Port=2
  nu : Inport  Port=3
  CentroidalMomentum : WBToolboxLibrary/Model/Dynamics/CentroidalMomentum
      settings: SourceProductName=WholeBodyToolbox
  "CoM6D ->  CoMXYZ1" : Selector  InputPortWidth=6+ROBOT_DOF  IndexOptions=Index vector (dialog)  Indices=[7:6+ROBOT_DOF]  OutputSizes=1
  "CoM6D ->  CoMXYZ2" : Selector  InputPortWidth=6+ROBOT_DOF  IndexOptions=Index vector (dialog)  Indices=[1 2 3 4 5 6]  OutputSizes=1
  GetBiasForces : WBToolboxLibrary/Model/Dynamics/GetBiasForces
      settings: SourceProductName=WholeBodyToolbox
  MassMatrix : WBToolboxLibrary/Model/Dynamics/MassMatrix
      settings: SourceProductName=WholeBodyToolbox
  M : Outport
  h : Outport  Port=2
  L : Outport  Port=3
  wires:
  CentroidalMomentum/1 -> L/1
  GetBiasForces/1 -> h/1
  w_H_b/1 -> CentroidalMomentum/1, GetBiasForces/1, MassMatrix/1
  jointPos/1 -> CentroidalMomentum/2, GetBiasForces/2, MassMatrix/2
  "CoM6D ->  CoMXYZ2"/1 -> CentroidalMomentum/3, GetBiasForces/3
  "CoM6D ->  CoMXYZ1"/1 -> CentroidalMomentum/4, GetBiasForces/4
  nu/1 -> "CoM6D ->  CoMXYZ1"/1, "CoM6D ->  CoMXYZ2"/1
  MassMatrix/1 -> M/1

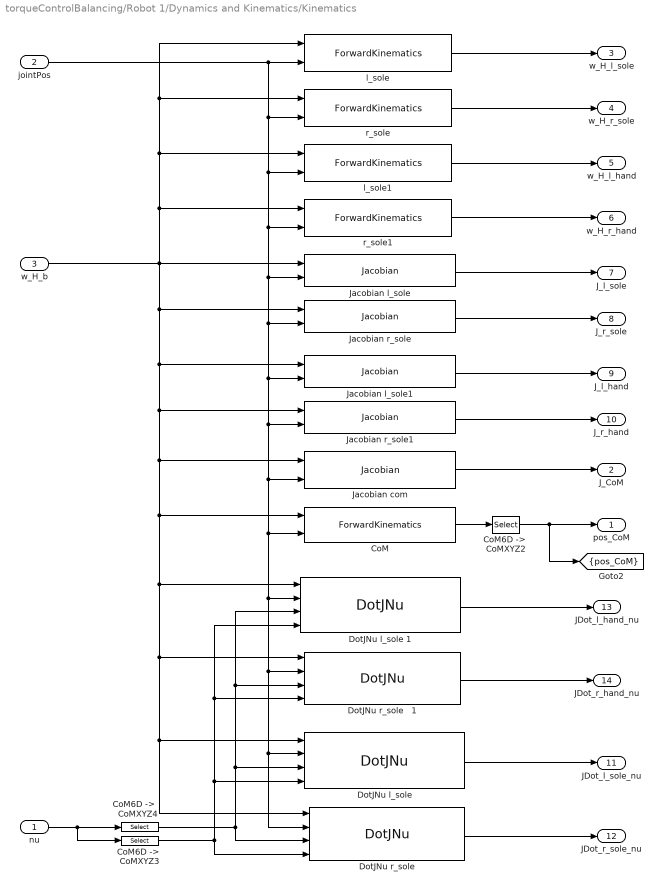
== system torqueControlBalancing/Robot 1/Dynamics and Kinematics/Kinematics ==
  nu : Inport
  jointPos : Inport  Port=2
  w_H_b : Inport  Port=3
  CoM : WBToolboxLibrary/Model/Kinematics/ForwardKinematics  frameName=Frames.COM
      settings: SourceProductName=WholeBodyToolbox
  "CoM6D ->  CoMXYZ2" : Selector  NumberOfDimensions=2  InputPortWidth=7  IndexOptions=Index vector (dialog),Index vector (dialog)  Indices=[1 2 3],[4]  OutputSizes=1,1
  "CoM6D ->  CoMXYZ3" : Selector  InputPortWidth=6+ROBOT_DOF  IndexOptions=Index vector (dialog)  Indices=[7:6+ROBOT_DOF]  OutputSizes=1
  "CoM6D ->  CoMXYZ4" : Selector  InputPortWidth=6+ROBOT_DOF  IndexOptions=Index vector (dialog)  Indices=[1 2 3 4 5 6]  OutputSizes=1
  "DotJNu l_sole " : WBToolboxLibrary/Model/Jacobians/DotJNu  frameName=Frames.LEFT_FOOT
      settings: SourceProductName=WholeBodyToolbox
  DotJNu l_sole 1 : WBToolboxLibrary/Model/Jacobians/DotJNu  frameName=Frames.LEFT_HAND
      settings: SourceProductName=WholeBodyToolbox
  "DotJNu r_sole   " : WBToolboxLibrary/Model/Jacobians/DotJNu  frameName=Frames.RIGHT_FOOT
      settings: SourceProductName=WholeBodyToolbox
  DotJNu r_sole   1 : WBToolboxLibrary/Model/Jacobians/DotJNu  frameName=Frames.RIGHT_HAND
      settings: SourceProductName=WholeBodyToolbox
  Jacobian com : WBToolboxLibrary/Model/Jacobians/Jacobian  frameName=Frames.COM
      settings: SourceProductName=WholeBodyToolbox
  Jacobian l_sole : WBToolboxLibrary/Model/Jacobians/Jacobian  frameName=Frames.LEFT_FOOT
      settings: SourceProductName=WholeBodyToolbox
  Jacobian l_sole1 : WBToolboxLibrary/Model/Jacobians/Jacobian  frameName=Frames.LEFT_HAND
      settings: SourceProductName=WholeBodyToolbox
  Jacobian r_sole : WBToolboxLibrary/Model/Jacobians/Jacobian  frameName=Frames.RIGHT_FOOT
      settings: SourceProductName=WholeBodyToolbox
  Jacobian r_sole1 : WBToolboxLibrary/Model/Jacobians/Jacobian  frameName=Frames.RIGHT_HAND
      settings: SourceProductName=WholeBodyToolbox
  l_sole : WBToolboxLibrary/Model/Kinematics/ForwardKinematics  frameName=Frames.LEFT_FOOT
      settings: SourceProductName=WholeBodyToolbox
  l_sole1 : WBToolboxLibrary/Model/Kinematics/ForwardKinematics  frameName=Frames.LEFT_HAND
      settings: SourceProductName=WholeBodyToolbox
  r_sole : WBToolboxLibrary/Model/Kinematics/ForwardKinematics  frameName=Frames.RIGHT_FOOT
      settings: SourceProductName=WholeBodyToolbox
  r_sole1 : WBToolboxLibrary/Model/Kinematics/ForwardKinematics  frameName=Frames.RIGHT_HAND
      settings: SourceProductName=WholeBodyToolbox
  pos_CoM : Outport
  J_CoM : Outport  Port=2
  w_H_l_sole : Outport  Port=3
  w_H_r_sole : Outport  Port=4
  w_H_l_hand : Outport  Port=5
  w_H_r_hand : Outport  Port=6
  J_l_sole : Outport  Port=7
  J_r_sole : Outport  Port=8
  J_l_hand : Outport  Port=9
  J_r_hand : Outport  Port=10
  JDot_l_sole_nu : Outport  Port=11
  JDot_r_sole_nu : Outport  Port=12
  JDot_l_hand_nu : Outport  Port=13
  JDot_r_hand_nu : Outport  Port=14
  tag scope: pos_CoM=scoped
  wires:
  "CoM6D ->  CoMXYZ3"/1 -> "DotJNu r_sole   "/4, DotJNu l_sole 1/4, DotJNu r_sole   1/4, "DotJNu l_sole "/4
  "CoM6D ->  CoMXYZ4"/1 -> "DotJNu r_sole   "/3, DotJNu r_sole   1/3, DotJNu l_sole 1/3, "DotJNu l_sole "/3
  nu/1 -> "CoM6D ->  CoMXYZ3"/1, "CoM6D ->  CoMXYZ4"/1
  l_sole/1 -> w_H_l_sole/1
  r_sole/1 -> w_H_r_sole/1
  Jacobian l_sole/1 -> J_l_sole/1
  Jacobian r_sole/1 -> J_r_sole/1
  Jacobian com/1 -> J_CoM/1
  CoM/1 -> "CoM6D ->  CoMXYZ2"/1
  "DotJNu l_sole "/1 -> JDot_l_sole_nu/1
  "DotJNu r_sole   "/1 -> JDot_r_sole_nu/1
  "CoM6D ->  CoMXYZ2"/1 -> [pos_CoM], pos_CoM/1
  Jacobian l_sole1/1 -> J_l_hand/1
  Jacobian r_sole1/1 -> J_r_hand/1
  w_H_b/1 -> Jacobian l_sole1/1, Jacobian com/1, DotJNu l_sole 1/1, DotJNu r_sole   1/1, "DotJNu r_sole   "/1, "DotJNu l_sole "/1, CoM/1, Jacobian r_sole1/1, Jacobian r_sole/1, Jacobian l_sole/1, r_sole1/1, l_sole1/1, r_sole/1, l_sole/1
  r_sole1/1 -> w_H_r_hand/1
  l_sole1/1 -> w_H_l_hand/1
  jointPos/1 -> l_sole1/2, r_sole1/2, Jacobian l_sole1/2, Jacobian r_sole1/2, Jacobian com/2, DotJNu l_sole 1/2, DotJNu r_sole   1/2, "DotJNu r_sole   "/2, "DotJNu l_sole "/2, CoM/2, Jacobian r_sole/2, Jacobian l_sole/2, r_sole/2, l_sole/2
  DotJNu r_sole   1/1 -> JDot_r_hand_nu/1
  DotJNu l_sole 1/1 -> JDot_l_hand_nu/1

== system torqueControlBalancing/Robot 1/Robot State and References/Compute State Velocity ==
  jointPos : Inport
  jointVel : Inport  Port=2
  w_H_b : Inport  Port=3
  Compute Base Velocity : MATLAB Function  TreatAsAtomicUnit=on
  Feet Jacobians : Subsystem
  Mux : Mux  Inputs=2
  nu : Outport
  wires:
  jointVel/1 -> Mux/2, Compute Base Velocity/3(jointVel)
  Mux/1 -> nu/1
  Compute Base Velocity/1(nu_b) -> Mux/1
  jointPos/1 -> Feet Jacobians/1(jointPos)
  w_H_b/1 -> Feet Jacobians/2(w_H_b)
  Feet Jacobians/1(J_l_sole) -> Compute Base Velocity/1(J_l_sole)
  Feet Jacobians/2(J_r_sole) -> Compute Base Velocity/2(J_r_sole)

== system torqueControlBalancing/Robot 1/Robot State and References/Compute base to fixed link transform ==
  jointPos : Inport
  Constant7 : Constant  Value=eye(4)
  "LFoot to base link transform " : Subsystem
  Relative transform l_sole_H_base : WBToolboxLibrary/Model/Kinematics/ForwardKinematics  frameName=Frames.LEFT_FOOT
      settings: SourceProductName=WholeBodyToolbox
  fixed_l_sole_H_b : Outport
  tag scope: jointPos=scoped
  wires:
  Constant7/1 -> "LFoot to base link transform "/3(w_H_base_fixed), Relative transform l_sole_H_base/1
  "LFoot to base link transform "/1(link_H_b) -> fixed_l_sole_H_b/1
  Relative transform l_sole_H_base/1 -> "LFoot to base link transform "/2(w_H_link)
  jointPos/1 -> [jointPos], "LFoot to base link transform "/1(jointPos), Relative transform l_sole_H_base/2

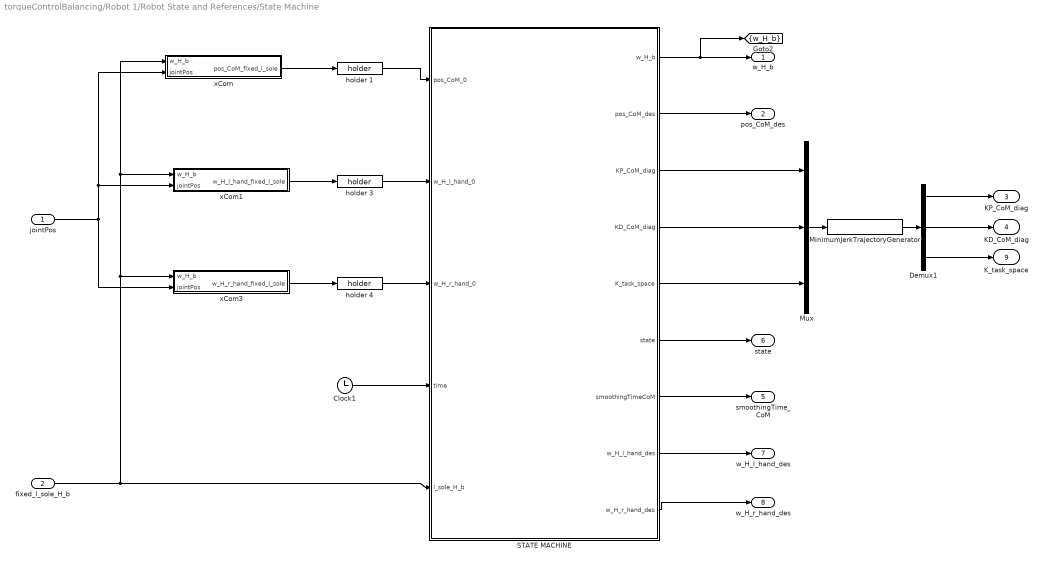
== system torqueControlBalancing/Robot 1/Robot State and References/State Machine ==
  jointPos : Inport
  fixed_l_sole_H_b : Inport  Port=2
  Clock1 : Clock
  Demux1 : Demux  Outputs=[3,3,2]
  MinimumJerkTrajectoryGenerator : WBToolboxLibrary/Utilities/MinimumJerkTrajectoryGenerator  externalSettlingTime=off  settlingTime=Config.SmoothingTimeGainScheduling  sampleTime=Config.tStep  resetOnSettlingTime=off  firstDerivatives=off  secondDerivatives=off  explicitInitialValue=off
      settings: SourceProductName=WholeBodyToolbox
  Mux : Mux  Inputs=3
  STATE MACHINE : MATLAB Function  TreatAsAtomicUnit=on
  holder 1 : WBToolboxLibrary/Utilities/holder 
      settings: SourceProductName=WholeBodyToolbox
  holder 3 : WBToolboxLibrary/Utilities/holder 
      settings: SourceProductName=WholeBodyToolbox
  holder 4 : WBToolboxLibrary/Utilities/holder 
      settings: SourceProductName=WholeBodyToolbox
  xCom : Subsystem
  xCom1 : Subsystem
  xCom3 : Subsystem
  w_H_b : Outport
  pos_CoM_des : Outport  Port=2
  KP_CoM_diag : Outport  Port=3
  KD_CoM_diag : Outport  Port=4
  smoothingTime_CoM : Outport  Port=5
  state : Outport  Port=6
  w_H_l_hand_des : Outport  Port=7
  w_H_r_hand_des : Outport  Port=8
  K_task_space : Outport  Port=9
  tag scope: w_H_b=scoped
  wires:
  xCom/1("pos_CoM_fixed_l_sole ") -> holder 1/1
  STATE MACHINE/2(pos_CoM_des) -> pos_CoM_des/1
  STATE MACHINE/6(state) -> state/1
  STATE MACHINE/3(KP_CoM_diag) -> Mux/1
  STATE MACHINE/4(KD_CoM_diag) -> Mux/2
  Mux/1 -> MinimumJerkTrajectoryGenerator/1
  MinimumJerkTrajectoryGenerator/1 -> Demux1/1
  jointPos/1 -> xCom1/2(jointPos), xCom/2(jointPos), xCom3/2(jointPos)
  fixed_l_sole_H_b/1 -> xCom/1(w_H_b), xCom1/1(w_H_b), xCom3/1(w_H_b), STATE MACHINE/5(l_sole_H_b)
  Clock1/1 -> STATE MACHINE/4(time)
  holder 1/1 -> STATE MACHINE/1(pos_CoM_0)
  STATE MACHINE/7(smoothingTimeCoM) -> smoothingTime_CoM/1
  STATE MACHINE/1(w_H_b) -> [w_H_b], w_H_b/1
  xCom1/1("w_H_l_hand_fixed_l_sole ") -> holder 3/1
  holder 3/1 -> STATE MACHINE/2(w_H_l_hand_0)
  xCom3/1("w_H_r_hand_fixed_l_sole ") -> holder 4/1
  holder 4/1 -> STATE MACHINE/3(w_H_r_hand_0)
  STATE MACHINE/5(K_task_space) -> Mux/3
  STATE MACHINE/8(w_H_l_hand_des) -> w_H_l_hand_des/1
  STATE MACHINE/9(w_H_r_hand_des) -> w_H_r_hand_des/1
  Demux1/1 -> KP_CoM_diag/1
  Demux1/2 -> KD_CoM_diag/1
  Demux1/3 -> K_task_space/1

== system torqueControlBalancing/Robot 1/Robot State and References/Update Gains and References ==
  pos_CoM_des : Inport
  KP_CoM_diag : Inport  Port=2
  KD_CoM_diag : Inport  Port=3
  smoothingTime_CoM : Inport  Port=4
  Reshape Gains Matrices : Subsystem
  Selector1 : Selector  NumberOfDimensions=2  InputPortWidth=3  IndexOptions=Index vector (dialog),Index vector (dialog)  Indices=[1 2 3],[1]  OutputSizes=1,1
  Smooth reference CoM : Subsystem
  KP_CoM : Outport
  KD_CoM : Outport  Port=2
  desired_pos_vel_acc_CoM : Outport  Port=3
  tag scope: pos_CoM_des=scoped
  wires:
  pos_CoM_des/1 -> Smooth reference CoM/1(pos_CoM_des)
  smoothingTime_CoM/1 -> Smooth reference CoM/2(smoothingTime_CoM)
  Smooth reference CoM/1(desired_pos_vel_acc_CoM) -> Selector1/1, desired_pos_vel_acc_CoM/1
  KP_CoM_diag/1 -> Reshape Gains Matrices/1(KP_CoM_diag)
  KD_CoM_diag/1 -> Reshape Gains Matrices/2(KD_CoM_diag)
  Reshape Gains Matrices/1(KP_CoM) -> KP_CoM/1
  Reshape Gains Matrices/2(KD_CoM) -> KD_CoM/1
  Selector1/1 -> [pos_CoM_des]

== system torqueControlBalancing/Robot 1/emergency stop: joint limits/STOP IF JOINTS HIT THE LIMITS ==
  jointPos : Inport
  Enable : EnablePort
  Assertion : Assertion
  GetLimits : WBToolboxLibrary/States/GetLimits  limitsSource=ControlBoard  limitsType=Position
      settings: SourceProductName=WholeBodyToolbox
  MATLAB Function : MATLAB Function  TreatAsAtomicUnit=on
  index1 : Constant  Value=0.01  VectorParams1D=off
  wires:
  jointPos/1 -> MATLAB Function/3(u)
  MATLAB Function/1(inRange) -> Assertion/1
  GetLimits/1 -> MATLAB Function/1(umin)
  GetLimits/2 -> MATLAB Function/2(umax)
  index1/1 -> MATLAB Function/4(tol)

== system torqueControlBalancing/Robot 1/emergency stop: joint limits/STOP IF THERE ARE SPIKES IN THE ENCODERS ==
  jointPos : Inport
  Enable : EnablePort
  Assertion : Assertion
  MATLAB Function : MATLAB Function  TreatAsAtomicUnit=on
  index1 : Constant  Value=Sat.maxJointsPositionDelta  VectorParams1D=off
  wires:
  jointPos/1 -> MATLAB Function/1(u)
  MATLAB Function/1(noSpikes) -> Assertion/1
  index1/1 -> MATLAB Function/2(delta_u_max)

== system torqueControlBalancing/Robot 2/Balancing Controller QP/Compute Desired Torques ==
  HessianMatrixTwoFeet : Inport
  gradientTwoFeet : Inport  Port=2
  ConstraintsMatrixTwoFeet : Inport  Port=3
  bVectorConstraintsTwoFeet : Inport  Port=4
  tauModel : Inport  Port=5
  Sigma : Inport  Port=6
  Na : Inport  Port=7
  f_LDot : Inport  Port=8
  Add : Sum
  Add1 : Sum
  Product1 : Product  Multiplication=Matrix(*)
  Product2 : Product  Multiplication=Matrix(*)
  QPSolver : Subsystem
  tau_QP : Outport
  wires:
  Na/1 -> Product2/1
  Product1/1 -> Add/2
  tauModel/1 -> Add/1
  Add/1 -> tau_QP/1
  Add1/1 -> Product1/2
  f_LDot/1 -> Add1/1
  Product2/1 -> Add1/2
  Sigma/1 -> Product1/1
  QPSolver/1(f_0_twoFeet) -> Product2/2
  ConstraintsMatrixTwoFeet/1 -> QPSolver/3(ConstraintsMatrixTwoFeet)
  gradientTwoFeet/1 -> QPSolver/2(gradientTwoFeet)
  HessianMatrixTwoFeet/1 -> QPSolver/1(HessianMatrixTwoFeet)
  bVectorConstraintsTwoFeet/1 -> QPSolver/4(bVectorConstraintsTwoFeet)

== system torqueControlBalancing/Robot 2/Dump and visualize/Visualize eventual QP failures ==
  QPStatus : Inport
  state : Inport  Port=2
  Enable : EnablePort
  QP status (0: no failure) : Scope  NumInputPorts=2
  wires:
  QPStatus/1 -> QP status (0: no failure)/1
  state/1 -> QP status (0: no failure)/2
